simulink model "plant"  (R2026a)
settings: Solver=VariableStepAuto  StopTime=11
InitFcn:
  | run('plant_parameters.m');
values from neighbouring files (symbols this model uses):
  d = 0.1845    [plant_parameters.m]
  dd = d / sqrt(2)    [plant_parameters.m]
  Kd_J1 = 40    [plant_parameters.m]
  Kd_J2 = 30    [plant_parameters.m]
  Kd_J3 = 12    [plant_parameters.m]
  Ki_J1 = 800    [plant_parameters.m]
  Ki_J2 = 700    [plant_parameters.m]
  Ki_J3 = 300    [plant_parameters.m]
  Kp_J1 = 800    [plant_parameters.m]
  Kp_J2 = 600    [plant_parameters.m]
  Kp_J3 = 250    [plant_parameters.m]
  L1 = 0.074    [plant_parameters.m]
  L2 = 0.121    [plant_parameters.m]
  L3 = 0.230    (= 0.23)    [plant_parameters.m]
  N_J1 = 120    [plant_parameters.m]
  N_J2 = 120    [plant_parameters.m]
  N_J3 = 120    [plant_parameters.m]
  Sampling_Time = 0.005    [plant_parameters.m]
undefined symbols (not defined in the file or in its folder): X, Y, Z
libraries: sm_lib x121, nesl_utility x55, slpidlib x18
(part 1 of 8)
settings Model: Creator=bogon  LastModifiedBy=bogon

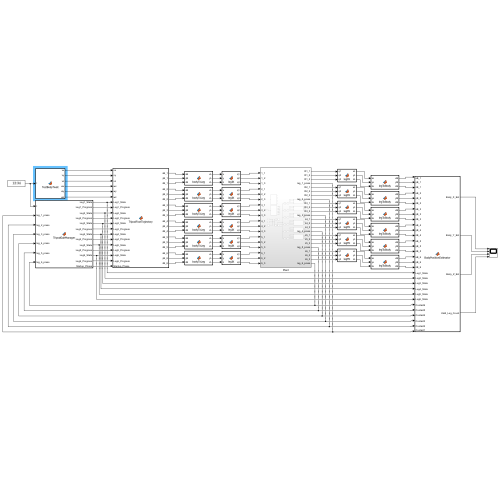
[thumbnail: Simulink's stored preview of the top-level diagram]
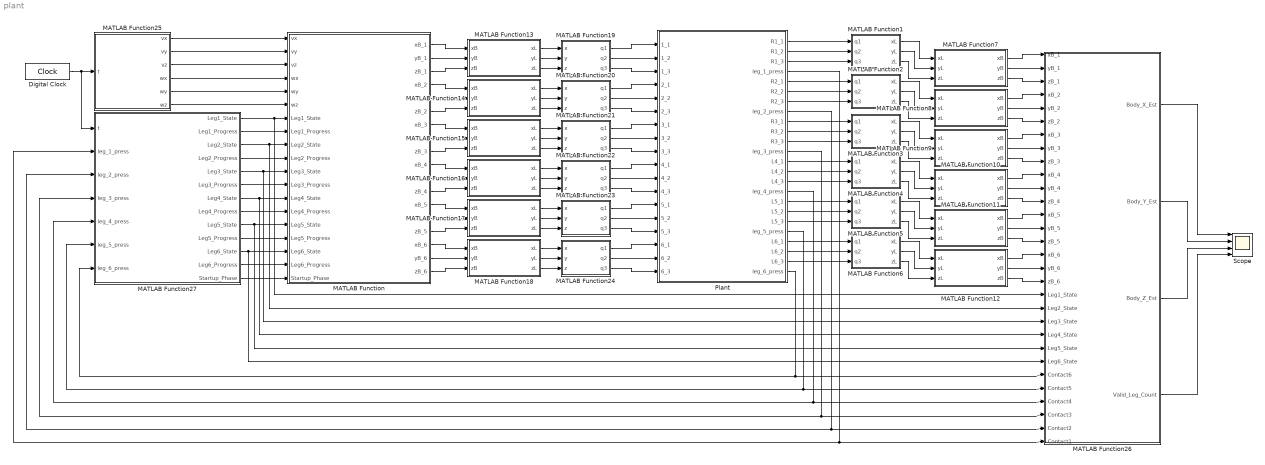
== system plant ==
  Digital Clock : DigitalClock  SampleTime=Sampling_Time
  MATLAB Function : MATLAB Function  TreatAsAtomicUnit=on
  MATLAB Function1 : MATLAB Function  TreatAsAtomicUnit=on
  MATLAB Function10 : MATLAB Function  TreatAsAtomicUnit=on
  MATLAB Function11 : MATLAB Function  TreatAsAtomicUnit=on
  MATLAB Function12 : MATLAB Function  TreatAsAtomicUnit=on
  MATLAB Function13 : MATLAB Function  TreatAsAtomicUnit=on
  MATLAB Function14 : MATLAB Function  TreatAsAtomicUnit=on
  MATLAB Function15 : MATLAB Function  TreatAsAtomicUnit=on
  MATLAB Function16 : MATLAB Function  TreatAsAtomicUnit=on
  MATLAB Function17 : MATLAB Function  TreatAsAtomicUnit=on
  MATLAB Function18 : MATLAB Function  TreatAsAtomicUnit=on
  MATLAB Function19 : MATLAB Function  TreatAsAtomicUnit=on
  MATLAB Function2 : MATLAB Function  TreatAsAtomicUnit=on
  MATLAB Function20 : MATLAB Function  TreatAsAtomicUnit=on
  MATLAB Function21 : MATLAB Function  TreatAsAtomicUnit=on
  MATLAB Function22 : MATLAB Function  TreatAsAtomicUnit=on
  MATLAB Function23 : MATLAB Function  TreatAsAtomicUnit=on
  MATLAB Function24 : MATLAB Function  TreatAsAtomicUnit=on
  MATLAB Function25 : MATLAB Function  TreatAsAtomicUnit=on
  MATLAB Function26 : MATLAB Function  TreatAsAtomicUnit=on  SystemSampleTime=Sampling_Time
  MATLAB Function27 : MATLAB Function  TreatAsAtomicUnit=on
  MATLAB Function3 : MATLAB Function  TreatAsAtomicUnit=on
  MATLAB Function4 : MATLAB Function  TreatAsAtomicUnit=on
  MATLAB Function5 : MATLAB Function  TreatAsAtomicUnit=on
  MATLAB Function6 : MATLAB Function  TreatAsAtomicUnit=on
  MATLAB Function7 : MATLAB Function  TreatAsAtomicUnit=on
  MATLAB Function8 : MATLAB Function  TreatAsAtomicUnit=on
  MATLAB Function9 : MATLAB Function  TreatAsAtomicUnit=on
  Plant : Subsystem
  Scope : Scope  NumInputPorts=4
      settings: ActiveDisplayYMinimum=-3.1042012313067247  ActiveDisplayYMaximum=1.7303656403267551
  wires:
  Plant/1(R1_1) -> MATLAB Function1/1(q1)
  Plant/2(R1_2) -> MATLAB Function1/2(q2)
  Plant/3(R1_3) -> MATLAB Function1/3(q3)
  Plant/9(R3_1) -> MATLAB Function3/1(q1)
  Plant/10(R3_2) -> MATLAB Function3/2(q2)
  Plant/11(R3_3) -> MATLAB Function3/3(q3)
  Plant/5(R2_1) -> MATLAB Function2/1(q1)
  Plant/6(R2_2) -> MATLAB Function2/2(q2)
  Plant/7(R2_3) -> MATLAB Function2/3(q3)
  Plant/13(L4_1) -> MATLAB Function4/1(q1)
  Plant/14(L4_2) -> MATLAB Function4/2(q2)
  Plant/15(L4_3) -> MATLAB Function4/3(q3)
  Plant/17(L5_1) -> MATLAB Function5/1(q1)
  Plant/18(L5_2) -> MATLAB Function5/2(q2)
  Plant/19(L5_3) -> MATLAB Function5/3(q3)
  Plant/21(L6_1) -> MATLAB Function6/1(q1)
  Plant/22(L6_2) -> MATLAB Function6/2(q2)
  Plant/23(L6_3) -> MATLAB Function6/3(q3)
  MATLAB Function16/1(xL) -> MATLAB Function22/1(x)
  MATLAB Function16/3(zL) -> MATLAB Function22/3(z)
  MATLAB Function16/2(yL) -> MATLAB Function22/2(y)
  MATLAB Function18/1(xL) -> MATLAB Function24/1(x)
  MATLAB Function17/3(zL) -> MATLAB Function23/3(z)
  MATLAB Function17/1(xL) -> MATLAB Function23/1(x)
  MATLAB Function18/2(yL) -> MATLAB Function24/2(y)
  MATLAB Function17/2(yL) -> MATLAB Function23/2(y)
  MATLAB Function14/3(zL) -> MATLAB Function20/3(z)
  MATLAB Function13/2(yL) -> MATLAB Function19/2(y)
  MATLAB Function15/3(zL) -> MATLAB Function21/3(z)
  MATLAB Function18/3(zL) -> MATLAB Function24/3(z)
  MATLAB Function/14(yB_5) -> MATLAB Function17/2(yB)
  MATLAB Function15/2(yL) -> MATLAB Function21/2(y)
  MATLAB Function/18(zB_6) -> MATLAB Function18/3(zB)
  MATLAB Function/5(yB_2) -> MATLAB Function14/2(yB)
  MATLAB Function/16(xB_6) -> MATLAB Function18/1(xB)
  MATLAB Function/17(yB_6) -> MATLAB Function18/2(yB)
  MATLAB Function/6(zB_2) -> MATLAB Function14/3(zB)
  MATLAB Function/11(yB_4) -> MATLAB Function16/2(yB)
  MATLAB Function/13(xB_5) -> MATLAB Function17/1(xB)
  MATLAB Function/8(yB_3) -> MATLAB Function15/2(yB)
  MATLAB Function/15(zB_5) -> MATLAB Function17/3(zB)
  MATLAB Function14/1(xL) -> MATLAB Function20/1(x)
  MATLAB Function/10(xB_4) -> MATLAB Function16/1(xB)
  MATLAB Function/4(xB_2) -> MATLAB Function14/1(xB)
  MATLAB Function/9(zB_3) -> MATLAB Function15/3(zB)
  MATLAB Function14/2(yL) -> MATLAB Function20/2(y)
  MATLAB Function/12(zB_4) -> MATLAB Function16/3(zB)
  MATLAB Function/7(xB_3) -> MATLAB Function15/1(xB)
  MATLAB Function13/3(zL) -> MATLAB Function19/3(z)
  MATLAB Function15/1(xL) -> MATLAB Function21/1(x)
  MATLAB Function13/1(xL) -> MATLAB Function19/1(x)
  MATLAB Function19/1(q1) -> Plant/1(1_1)
  MATLAB Function19/2(q2) -> Plant/2(1_2)
  MATLAB Function19/3(q3) -> Plant/3(1_3)
  MATLAB Function20/2(q2) -> Plant/5(2_2)
  MATLAB Function20/1(q1) -> Plant/4(2_1)
  MATLAB Function20/3(q3) -> Plant/6(2_3)
  MATLAB Function21/1(q1) -> Plant/7(3_1)
  MATLAB Function21/2(q2) -> Plant/8(3_2)
  MATLAB Function21/3(q3) -> Plant/9(3_3)
  MATLAB Function22/1(q1) -> Plant/10(4_1)
  MATLAB Function22/2(q2) -> Plant/11(4_2)
  MATLAB Function22/3(q3) -> Plant/12(4_3)
  MATLAB Function23/1(q1) -> Plant/13(5_1)
  MATLAB Function23/2(q2) -> Plant/14(5_2)
  MATLAB Function23/3(q3) -> Plant/15(5_3)
  MATLAB Function24/2(q2) -> Plant/17(6_2)
  MATLAB Function24/1(q1) -> Plant/16(6_1)
  MATLAB Function24/3(q3) -> Plant/18(6_3)
  MATLAB Function1/1(xL) -> MATLAB Function7/1(xL)
  MATLAB Function1/2(yL) -> MATLAB Function7/2(yL)
  MATLAB Function1/3(zL) -> MATLAB Function7/3(zL)
  MATLAB Function2/1(xL) -> MATLAB Function8/1(xL)
  MATLAB Function2/2(yL) -> MATLAB Function8/2(yL)
  MATLAB Function2/3(zL) -> MATLAB Function8/3(zL)
  MATLAB Function3/1(xL) -> MATLAB Function9/1(xL)
  MATLAB Function3/2(yL) -> MATLAB Function9/2(yL)
  MATLAB Function3/3(zL) -> MATLAB Function9/3(zL)
  MATLAB Function4/1(xL) -> MATLAB Function10/1(xL)
  MATLAB Function4/2(yL) -> MATLAB Function10/2(yL)
  MATLAB Function4/3(zL) -> MATLAB Function10/3(zL)
  MATLAB Function5/1(xL) -> MATLAB Function11/1(xL)
  MATLAB Function5/2(yL) -> MATLAB Function11/2(yL)
  MATLAB Function5/3(zL) -> MATLAB Function11/3(zL)
  MATLAB Function6/1(xL) -> MATLAB Function12/1(xL)
  MATLAB Function6/2(yL) -> MATLAB Function12/2(yL)
  MATLAB Function6/3(zL) -> MATLAB Function12/3(zL)
  Digital Clock/1 -> MATLAB Function27/1(t), MATLAB Function25/1(t)
  MATLAB Function/1(xB_1) -> MATLAB Function13/1(xB)
  MATLAB Function/2(yB_1) -> MATLAB Function13/2(yB)
  MATLAB Function/3(zB_1) -> MATLAB Function13/3(zB)
  MATLAB Function25/1(vx) -> MATLAB Function/1(vx)
  MATLAB Function25/2(vy) -> MATLAB Function/2(vy)
  MATLAB Function25/3(vz) -> MATLAB Function/3(vz)
  MATLAB Function25/4(wx) -> MATLAB Function/4(wx)
  MATLAB Function25/5(wy) -> MATLAB Function/5(wy)
  MATLAB Function25/6(wz) -> MATLAB Function/6(wz)
  MATLAB Function27/1(Leg1_State) -> MATLAB Function26/19(Leg1_State), MATLAB Function/7(Leg1_State)
  MATLAB Function27/2(Leg1_Progress) -> MATLAB Function/8(Leg1_Progress)
  MATLAB Function27/3(Leg2_State) -> MATLAB Function26/20(Leg2_State), MATLAB Function/9(Leg2_State)
  MATLAB Function27/4(Leg2_Progress) -> MATLAB Function/10(Leg2_Progress)
  MATLAB Function27/5(Leg3_State) -> MATLAB Function26/21(Leg3_State), MATLAB Function/11(Leg3_State)
  MATLAB Function27/6(Leg3_Progress) -> MATLAB Function/12(Leg3_Progress)
  MATLAB Function27/7(Leg4_State) -> MATLAB Function26/22(Leg4_State), MATLAB Function/13(Leg4_State)
  MATLAB Function27/8(Leg4_Progress) -> MATLAB Function/14(Leg4_Progress)
  MATLAB Function27/9(Leg5_State) -> MATLAB Function26/23(Leg5_State), MATLAB Function/15(Leg5_State)
  MATLAB Function27/10(Leg5_Progress) -> MATLAB Function/16(Leg5_Progress)
  MATLAB Function27/11(Leg6_State) -> MATLAB Function26/24(Leg6_State), MATLAB Function/17(Leg6_State)
  MATLAB Function27/12(Leg6_Progress) -> MATLAB Function/18(Leg6_Progress)
  MATLAB Function27/13(Startup_Phase) -> MATLAB Function/19(Startup_Phase)
  Plant/4(leg_1_press) -> MATLAB Function26/30(Contact1), MATLAB Function27/2(leg_1_press)
  Plant/8(leg_2_press) -> MATLAB Function26/29(Contact2), MATLAB Function27/3(leg_2_press)
  Plant/12(leg_3_press) -> MATLAB Function27/4(leg_3_press), MATLAB Function26/28(Contact3)
  Plant/16(leg_4_press) -> MATLAB Function26/27(Contact4), MATLAB Function27/5(leg_4_press)
  Plant/20(leg_5_press) -> MATLAB Function27/6(leg_5_press), MATLAB Function26/26(Contact5)
  Plant/24(leg_6_press) -> MATLAB Function27/7(leg_6_press), MATLAB Function26/25(Contact6)
  MATLAB Function7/1(xB) -> MATLAB Function26/1(xB_1)
  MATLAB Function7/2(yB) -> MATLAB Function26/2(yB_1)
  MATLAB Function7/3(zB) -> MATLAB Function26/3(zB_1)
  MATLAB Function12/3(zB) -> MATLAB Function26/18(zB_6)
  MATLAB Function12/2(yB) -> MATLAB Function26/17(yB_6)
  MATLAB Function12/1(xB) -> MATLAB Function26/16(xB_6)
  MATLAB Function8/2(yB) -> MATLAB Function26/5(yB_2)
  MATLAB Function9/2(yB) -> MATLAB Function26/8(yB_3)
  MATLAB Function10/2(yB) -> MATLAB Function26/11(yB_4)
  MATLAB Function11/2(yB) -> MATLAB Function26/14(yB_5)
  MATLAB Function11/3(zB) -> MATLAB Function26/15(zB_5)
  MATLAB Function11/1(xB) -> MATLAB Function26/13(xB_5)
  MATLAB Function10/3(zB) -> MATLAB Function26/12(zB_4)
  MATLAB Function10/1(xB) -> MATLAB Function26/10(xB_4)
  MATLAB Function9/3(zB) -> MATLAB Function26/9(zB_3)
  MATLAB Function9/1(xB) -> MATLAB Function26/7(xB_3)
  MATLAB Function8/3(zB) -> MATLAB Function26/6(zB_2)
  MATLAB Function8/1(xB) -> MATLAB Function26/4(xB_2)
  MATLAB Function26/1(Body_X_Est) -> Scope/1
  MATLAB Function26/2(Body_Y_Est) -> Scope/2
  MATLAB Function26/3(Body_Z_Est) -> Scope/3
  MATLAB Function26/4(Valid_Leg_Count) -> Scope/4

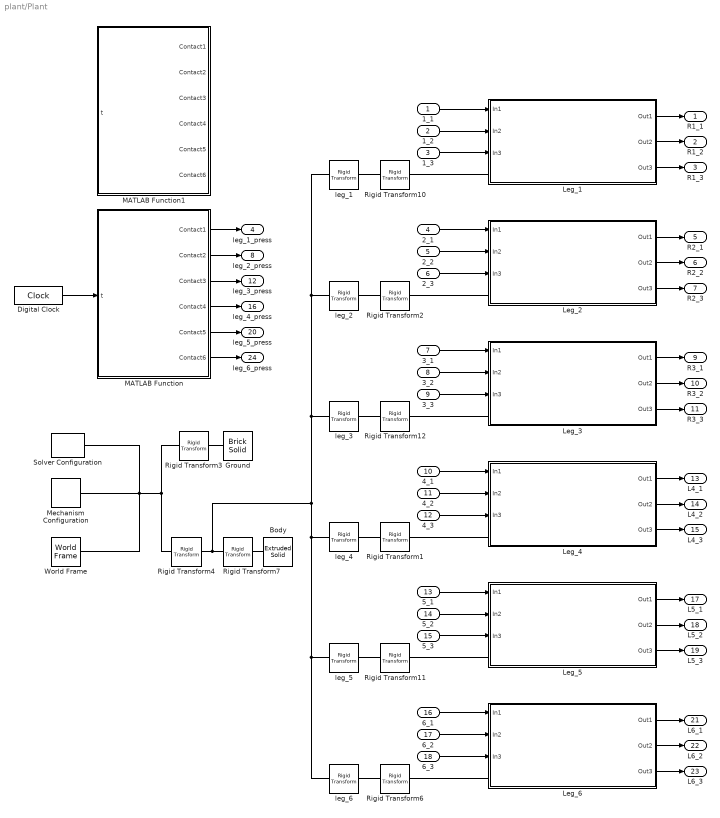
== system plant/Plant ==
  1_1 : Inport
  1_2 : Inport  Port=2
  1_3 : Inport  Port=3
  2_1 : Inport  Port=4
  2_2 : Inport  Port=5
  2_3 : Inport  Port=6
  3_1 : Inport  Port=7
  3_2 : Inport  Port=8
  3_3 : Inport  Port=9
  4_1 : Inport  Port=10
  4_2 : Inport  Port=11
  4_3 : Inport  Port=12
  5_1 : Inport  Port=13
  5_2 : Inport  Port=14
  5_3 : Inport  Port=15
  6_1 : Inport  Port=16
  6_2 : Inport  Port=17
  6_3 : Inport  Port=18
  Body : sm_lib/Body Elements/Extruded Solid  ExtrusionType=Regular  PolygonNumSides=8  PolygonOuterRadius=Body_r  PolygonOuterRadiusUnits=m  ExportEntireGeometry=off  ExtrusionCrossSection=[1 1; -1 1; -1 -1; 1 -1]  ExtrusionCrossSectionUnits=m  ExportConvexHullGeometry=off  ExtrusionLength=Body_t  ExtrusionLengthUnits=m  InertiaType=CalculateFromGeometry  BasedOnType=Density  Density=1000  DensityUnits=kg/m^3  Mass=1  MassUnits=kg  CenterOfMass=[0 0 0]  CenterOfMassUnits=m  MomentsOfInertia=[1 1 1]  MomentsOfInertiaUnits=kg*m^2  ProductsOfInertia=[0 0 0]  ProductsOfInertiaUnits=kg*m^2  GraphicType=FromGeometry  MarkerShape=Sphere  MarkerSize=10  GraphicVisPropType=SimpleVisualProperties  GraphicDiffuseColor=[0 0 0]  GraphicOpacity=1  GraphicSpecularColor=[0.5 0.5 0.5 1.0]  GraphicAmbientColor=[0.15 0.15 0.15 1.0]  GraphicEmissiveColor=[0.0 0.0 0.0 1.0]  GraphicShininess=75  DoExposeReferenceFrame=on  SerializedFrames=<Frames/>
  Digital Clock : DigitalClock  SampleTime=Sampling_Time
  Ground : sm_lib/Body Elements/Brick Solid  BrickDimensions=[2 2 0.05]  BrickDimensionsUnits=m  ExportEntireGeometry=off  InertiaType=CalculateFromGeometry  BasedOnType=Density  Density=1000  DensityUnits=kg/m^3  Mass=1  MassUnits=kg  CenterOfMass=[0 0 0]  CenterOfMassUnits=m  MomentsOfInertia=[1 1 1]  MomentsOfInertiaUnits=kg*m^2  ProductsOfInertia=[0 0 0]  ProductsOfInertiaUnits=kg*m^2  GraphicType=FromGeometry  MarkerShape=Sphere  MarkerSize=10  GraphicVisPropType=SimpleVisualProperties  GraphicDiffuseColor=[0 1 0.498]  GraphicOpacity=1  GraphicSpecularColor=[0.5 0.5 0.5 1.0]  GraphicAmbientColor=[0.15 0.15 0.15 1.0]  GraphicEmissiveColor=[0.0 0.0 0.0 1.0]  GraphicShininess=75  DoExposeReferenceFrame=on  SerializedFrames=<Frames/>
  Leg_1 : Subsystem
  Leg_2 : Subsystem
  Leg_3 : Subsystem
  Leg_4 : Subsystem
  Leg_5 : Subsystem
  Leg_6 : Subsystem
  MATLAB Function : MATLAB Function  TreatAsAtomicUnit=on
  MATLAB Function1 : MATLAB Function  TreatAsAtomicUnit=on
  Mechanism Configuration : sm_lib/Utilities/Mechanism Configuration  UniformGravity=Constant  GravityVector=[0 0 -9.80665]  GravityVectorUnits=m/s^2  LinearizationDelta=0.001  JointModeTransitionNonlinearIterations=2
  Rigid Transform1 : sm_lib/Frames and Transforms/Rigid Transform  RotationMethod=StandardAxis  FollAlignAxisA=+X  BaseAlignAxisA=+Y  FollAlignAxisB=+Y  BaseAlignAxisB=+Z  RotationStandardAxis=+Z  RotationAngle=45  RotationAngleUnits=deg  RotationArbitraryAxis=[0 0 1]  RotationSequenceAxes=FollowerAxes  RotationSequence=XYX  RotationSequenceAngles=[0 0 0]  RotationSequenceAnglesUnits=deg  RotationMatrix=[1 0 0;0 1 0;0 0 1]  Quaternion=[1 0 0 0]  TranslationMethod=None  TranslationCartesianOffset=[0 0 -0.025]  TranslationCartesianOffsetUnits=m  TranslationStandardAxis=-Z  TranslationStandardOffset=0.025  TranslationStandardOffsetUnits=m  TranslationROffset=0  TranslationROffsetUnits=m  TranslationThetaOffset=0  TranslationThetaOffsetUnits=deg  TranslationZOffset=0  TranslationZOffsetUnits=m
  Rigid Transform10 : sm_lib/Frames and Transforms/Rigid Transform  RotationMethod=StandardAxis  FollAlignAxisA=+X  BaseAlignAxisA=+Y  FollAlignAxisB=+Y  BaseAlignAxisB=+Z  RotationStandardAxis=-Z  RotationAngle=45  RotationAngleUnits=deg  RotationArbitraryAxis=[0 0 1]  RotationSequenceAxes=FollowerAxes  RotationSequence=XYX  RotationSequenceAngles=[0 0 0]  RotationSequenceAnglesUnits=deg  RotationMatrix=[1 0 0;0 1 0;0 0 1]  Quaternion=[1 0 0 0]  TranslationMethod=None  TranslationCartesianOffset=[0 0 -0.025]  TranslationCartesianOffsetUnits=m  TranslationStandardAxis=-Z  TranslationStandardOffset=0.025  TranslationStandardOffsetUnits=m  TranslationROffset=0  TranslationROffsetUnits=m  TranslationThetaOffset=0  TranslationThetaOffsetUnits=deg  TranslationZOffset=0  TranslationZOffsetUnits=m
  Rigid Transform11 : sm_lib/Frames and Transforms/Rigid Transform  RotationMethod=StandardAxis  FollAlignAxisA=+X  BaseAlignAxisA=+Y  FollAlignAxisB=+Y  BaseAlignAxisB=+Z  RotationStandardAxis=+Z  RotationAngle=90  RotationAngleUnits=deg  RotationArbitraryAxis=[0 0 1]  RotationSequenceAxes=FollowerAxes  RotationSequence=XYX  RotationSequenceAngles=[0 0 0]  RotationSequenceAnglesUnits=deg  RotationMatrix=[1 0 0;0 1 0;0 0 1]  Quaternion=[1 0 0 0]  TranslationMethod=None  TranslationCartesianOffset=[0 0 -0.025]  TranslationCartesianOffsetUnits=m  TranslationStandardAxis=-Z  TranslationStandardOffset=0.025  TranslationStandardOffsetUnits=m  TranslationROffset=0  TranslationROffsetUnits=m  TranslationThetaOffset=0  TranslationThetaOffsetUnits=deg  TranslationZOffset=0  TranslationZOffsetUnits=m
  Rigid Transform12 : sm_lib/Frames and Transforms/Rigid Transform  RotationMethod=StandardAxis  FollAlignAxisA=+X  BaseAlignAxisA=+Y  FollAlignAxisB=+Y  BaseAlignAxisB=+Z  RotationStandardAxis=-Z  RotationAngle=135  RotationAngleUnits=deg  RotationArbitraryAxis=[0 0 1]  RotationSequenceAxes=BaseAxes  RotationSequence=XYX  RotationSequenceAngles=[0 0 0]  RotationSequenceAnglesUnits=deg  RotationMatrix=[1 0 0;0 1 0;0 0 1]  Quaternion=[1 0 0 0]  TranslationMethod=None  TranslationCartesianOffset=[0 0 -0.025]  TranslationCartesianOffsetUnits=m  TranslationStandardAxis=-Z  TranslationStandardOffset=0.025  TranslationStandardOffsetUnits=m  TranslationROffset=0  TranslationROffsetUnits=m  TranslationThetaOffset=0  TranslationThetaOffsetUnits=deg  TranslationZOffset=0  TranslationZOffsetUnits=m
  Rigid Transform2 : sm_lib/Frames and Transforms/Rigid Transform  RotationMethod=StandardAxis  FollAlignAxisA=+X  BaseAlignAxisA=+Y  FollAlignAxisB=+Y  BaseAlignAxisB=+Z  RotationStandardAxis=-Z  RotationAngle=90  RotationAngleUnits=deg  RotationArbitraryAxis=[0 0 1]  RotationSequenceAxes=FollowerAxes  RotationSequence=XYX  RotationSequenceAngles=[0 0 0]  RotationSequenceAnglesUnits=deg  RotationMatrix=[1 0 0;0 1 0;0 0 1]  Quaternion=[1 0 0 0]  TranslationMethod=None  TranslationCartesianOffset=[0 0 -0.025]  TranslationCartesianOffsetUnits=m  TranslationStandardAxis=-Z  TranslationStandardOffset=0.025  TranslationStandardOffsetUnits=m  TranslationROffset=0  TranslationROffsetUnits=m  TranslationThetaOffset=0  TranslationThetaOffsetUnits=deg  TranslationZOffset=0  TranslationZOffsetUnits=m
  Rigid Transform3 : sm_lib/Frames and Transforms/Rigid Transform  RotationMethod=None  FollAlignAxisA=+X  BaseAlignAxisA=+Y  FollAlignAxisB=+Y  BaseAlignAxisB=+Z  RotationStandardAxis=+Z  RotationAngle=0  RotationAngleUnits=deg  RotationArbitraryAxis=[0 0 1]  RotationSequenceAxes=FollowerAxes  RotationSequence=XYX  RotationSequenceAngles=[0 0 0]  RotationSequenceAnglesUnits=deg  RotationMatrix=[1 0 0;0 1 0;0 0 1]  Quaternion=[1 0 0 0]  TranslationMethod=Cartesian  TranslationCartesianOffset=[0 0 -0.025]  TranslationCartesianOffsetUnits=m  TranslationStandardAxis=-Z  TranslationStandardOffset=0.025  TranslationStandardOffsetUnits=m  TranslationROffset=0  TranslationROffsetUnits=m  TranslationThetaOffset=0  TranslationThetaOffsetUnits=deg  TranslationZOffset=0  TranslationZOffsetUnits=m
  Rigid Transform4 : sm_lib/Frames and Transforms/Rigid Transform  RotationMethod=None  FollAlignAxisA=+X  BaseAlignAxisA=+Y  FollAlignAxisB=+Y  BaseAlignAxisB=+Z  RotationStandardAxis=+Z  RotationAngle=90  RotationAngleUnits=deg  RotationArbitraryAxis=[0 0 1]  RotationSequenceAxes=FollowerAxes  RotationSequence=XYX  RotationSequenceAngles=[0 0 0]  RotationSequenceAnglesUnits=deg  RotationMatrix=[1 0 0;0 1 0;0 0 1]  Quaternion=[1 0 0 0]  TranslationMethod=StandardAxis  TranslationCartesianOffset=[0 0 0]  TranslationCartesianOffsetUnits=m  TranslationStandardAxis=+Z  TranslationStandardOffset=Reference_point  TranslationStandardOffsetUnits=m  TranslationROffset=0  TranslationROffsetUnits=m  TranslationThetaOffset=0  TranslationThetaOffsetUnits=deg  TranslationZOffset=0  TranslationZOffsetUnits=m
  Rigid Transform6 : sm_lib/Frames and Transforms/Rigid Transform  RotationMethod=StandardAxis  FollAlignAxisA=+X  BaseAlignAxisA=+Y  FollAlignAxisB=+Y  BaseAlignAxisB=+Z  RotationStandardAxis=+Z  RotationAngle=135  RotationAngleUnits=deg  RotationArbitraryAxis=[0 0 1]  RotationSequenceAxes=FollowerAxes  RotationSequence=XYX  RotationSequenceAngles=[0 0 0]  RotationSequenceAnglesUnits=deg  RotationMatrix=[1 0 0;0 1 0;0 0 1]  Quaternion=[1 0 0 0]  TranslationMethod=None  TranslationCartesianOffset=[0 0 -0.025]  TranslationCartesianOffsetUnits=m  TranslationStandardAxis=-Z  TranslationStandardOffset=0.025  TranslationStandardOffsetUnits=m  TranslationROffset=0  TranslationROffsetUnits=m  TranslationThetaOffset=0  TranslationThetaOffsetUnits=deg  TranslationZOffset=0  TranslationZOffsetUnits=m
  Rigid Transform7 : sm_lib/Frames and Transforms/Rigid Transform  RotationMethod=StandardAxis  FollAlignAxisA=+X  BaseAlignAxisA=+Y  FollAlignAxisB=+Y  BaseAlignAxisB=+Z  RotationStandardAxis=-Z  RotationAngle=22.5  RotationAngleUnits=deg  RotationArbitraryAxis=[0 0 1]  RotationSequenceAxes=FollowerAxes  RotationSequence=XYX  RotationSequenceAngles=[0 0 0]  RotationSequenceAnglesUnits=deg  RotationMatrix=[1 0 0;0 1 0;0 0 1]  Quaternion=[1 0 0 0]  TranslationMethod=None  TranslationCartesianOffset=[0 0 -0.025]  TranslationCartesianOffsetUnits=m  TranslationStandardAxis=+Y  TranslationStandardOffset=0.025  TranslationStandardOffsetUnits=m  TranslationROffset=0  TranslationROffsetUnits=m  TranslationThetaOffset=0  TranslationThetaOffsetUnits=deg  TranslationZOffset=0  TranslationZOffsetUnits=m
  Solver Configuration : nesl_utility/Solver Configuration  PhysicalDomain=network_engine_domain  SubClassName=solver  LeftPortType=input  RightPortType=generic  Tones=[]  Harmonics=[]  SimulateNoise=off  Profile=off  UseLocalSampling=off  EnableSwitchedLinearOptims=on  FrequencyDomain=off  UseCCode=off  RelTol=0.001  AbsTol=0.001  MinStep=1e-09  ToWorkspace=off  RevertToSquareIcSolve=off  NumHomotopyIterations=100  PhasorMode=off  PhasorModeNumHarmonics=1  ConsistencySolver=NEWTON_XTOL_AFTER_FTOL  CanonicalOrdering=CANONICAL  OptimizeIntermediates=OPTIMIZED  IndexReductionMethod=DerivativeReplacement  DoDC=off  ResidualTolerance=1e-09  ConsistencyTolSource=GLOBAL  ConsistencyAbsTol=0.001  ConsistencyRelTol=0.001  ConsistencyTolFactor=0.001  UseLocalSolver=off  LocalSolverChoice=NE_BACKWARD_EULER_ADVANCER  ResolveIndetEquations=on  FunctionEvalNumThread=1  LocalSolverSampleTime=0.001  DoFixedCost=off  MaxNonlinIter=3  MaxModeIter=2  ComputeImpulses=off  ImpulseIterations=2  LinearAlgebra=auto  LinearAlgebraNumThread=0  EquationFormulation=NE_TIME_EF  DelaysMemoryBudget=1024  AutomaticFiltering=on  FilteringTimeConstant=0.001  PartitionStorageMethod=AS_NEEDED  PartitionMemoryBudget=1024  PartitionMethod=ROBUST  MultibodyUseLocalSolver=off  MultibodyLocalSolverChoice=ODE1  MultibodyLocalSolverSampleTime=0.001
  World Frame : sm_lib/Frames and Transforms/World Frame
  leg_1 : sm_lib/Frames and Transforms/Rigid Transform  RotationMethod=None  FollAlignAxisA=+X  BaseAlignAxisA=+Y  FollAlignAxisB=+Y  BaseAlignAxisB=+Z  RotationStandardAxis=+Z  RotationAngle=0  RotationAngleUnits=deg  RotationArbitraryAxis=[0 0 1]  RotationSequenceAxes=FollowerAxes  RotationSequence=XYX  RotationSequenceAngles=[0 0 0]  RotationSequenceAnglesUnits=deg  RotationMatrix=[1 0 0;0 1 0;0 0 1]  Quaternion=[1 0 0 0]  TranslationMethod=Cartesian  TranslationCartesianOffset=[dd -dd 0]  TranslationCartesianOffsetUnits=m  TranslationStandardAxis=-Z  TranslationStandardOffset=0.025  TranslationStandardOffsetUnits=m  TranslationROffset=0  TranslationROffsetUnits=m  TranslationThetaOffset=0  TranslationThetaOffsetUnits=deg  TranslationZOffset=0  TranslationZOffsetUnits=m
  leg_2 : sm_lib/Frames and Transforms/Rigid Transform  RotationMethod=None  FollAlignAxisA=+X  BaseAlignAxisA=+Y  FollAlignAxisB=+Y  BaseAlignAxisB=+Z  RotationStandardAxis=+Z  RotationAngle=0  RotationAngleUnits=deg  RotationArbitraryAxis=[0 0 1]  RotationSequenceAxes=FollowerAxes  RotationSequence=XYX  RotationSequenceAngles=[0 0 0]  RotationSequenceAnglesUnits=deg  RotationMatrix=[1 0 0;0 1 0;0 0 1]  Quaternion=[1 0 0 0]  TranslationMethod=Cartesian  TranslationCartesianOffset=[0 -d 0]  TranslationCartesianOffsetUnits=m  TranslationStandardAxis=-Z  TranslationStandardOffset=0.025  TranslationStandardOffsetUnits=m  TranslationROffset=0  TranslationROffsetUnits=m  TranslationThetaOffset=0  TranslationThetaOffsetUnits=deg  TranslationZOffset=0  TranslationZOffsetUnits=m
  leg_3 : sm_lib/Frames and Transforms/Rigid Transform  RotationMethod=None  FollAlignAxisA=+X  BaseAlignAxisA=+Y  FollAlignAxisB=+Y  BaseAlignAxisB=+Z  RotationStandardAxis=+Z  RotationAngle=0  RotationAngleUnits=deg  RotationArbitraryAxis=[0 0 1]  RotationSequenceAxes=FollowerAxes  RotationSequence=XYX  RotationSequenceAngles=[0 0 0]  RotationSequenceAnglesUnits=deg  RotationMatrix=[1 0 0;0 1 0;0 0 1]  Quaternion=[1 0 0 0]  TranslationMethod=Cartesian  TranslationCartesianOffset=[-dd -dd 0]  TranslationCartesianOffsetUnits=m  TranslationStandardAxis=-Z  TranslationStandardOffset=0.025  TranslationStandardOffsetUnits=m  TranslationROffset=0  TranslationROffsetUnits=m  TranslationThetaOffset=0  TranslationThetaOffsetUnits=deg  TranslationZOffset=0  TranslationZOffsetUnits=m
  leg_4 : sm_lib/Frames and Transforms/Rigid Transform  RotationMethod=None  FollAlignAxisA=+X  BaseAlignAxisA=+Y  FollAlignAxisB=+Y  BaseAlignAxisB=+Z  RotationStandardAxis=+Z  RotationAngle=0  RotationAngleUnits=deg  RotationArbitraryAxis=[0 0 1]  RotationSequenceAxes=FollowerAxes  RotationSequence=XYX  RotationSequenceAngles=[0 0 0]  RotationSequenceAnglesUnits=deg  RotationMatrix=[1 0 0;0 1 0;0 0 1]  Quaternion=[1 0 0 0]  TranslationMethod=Cartesian  TranslationCartesianOffset=[dd dd 0]  TranslationCartesianOffsetUnits=m  TranslationStandardAxis=-Z  TranslationStandardOffset=0.025  TranslationStandardOffsetUnits=m  TranslationROffset=0  TranslationROffsetUnits=m  TranslationThetaOffset=0  TranslationThetaOffsetUnits=deg  TranslationZOffset=0  TranslationZOffsetUnits=m
  leg_5 : sm_lib/Frames and Transforms/Rigid Transform  RotationMethod=None  FollAlignAxisA=+X  BaseAlignAxisA=+Y  FollAlignAxisB=+Y  BaseAlignAxisB=+Z  RotationStandardAxis=+Z  RotationAngle=0  RotationAngleUnits=deg  RotationArbitraryAxis=[0 0 1]  RotationSequenceAxes=FollowerAxes  RotationSequence=XYX  RotationSequenceAngles=[0 0 0]  RotationSequenceAnglesUnits=deg  RotationMatrix=[1 0 0;0 1 0;0 0 1]  Quaternion=[1 0 0 0]  TranslationMethod=Cartesian  TranslationCartesianOffset=[0 d 0]  TranslationCartesianOffsetUnits=m  TranslationStandardAxis=-Z  TranslationStandardOffset=0.025  TranslationStandardOffsetUnits=m  TranslationROffset=0  TranslationROffsetUnits=m  TranslationThetaOffset=0  TranslationThetaOffsetUnits=deg  TranslationZOffset=0  TranslationZOffsetUnits=m
  leg_6 : sm_lib/Frames and Transforms/Rigid Transform  RotationMethod=None  FollAlignAxisA=+X  BaseAlignAxisA=+Y  FollAlignAxisB=+Y  BaseAlignAxisB=+Z  RotationStandardAxis=+Z  RotationAngle=0  RotationAngleUnits=deg  RotationArbitraryAxis=[0 0 1]  RotationSequenceAxes=FollowerAxes  RotationSequence=XYX  RotationSequenceAngles=[0 0 0]  RotationSequenceAnglesUnits=deg  RotationMatrix=[1 0 0;0 1 0;0 0 1]  Quaternion=[1 0 0 0]  TranslationMethod=Cartesian  TranslationCartesianOffset=[-dd dd 0]  TranslationCartesianOffsetUnits=m  TranslationStandardAxis=-Z  TranslationStandardOffset=0.025  TranslationStandardOffsetUnits=m  TranslationROffset=0  TranslationROffsetUnits=m  TranslationThetaOffset=0  TranslationThetaOffsetUnits=deg  TranslationZOffset=0  TranslationZOffsetUnits=m
  R1_1 : Outport
  R1_2 : Outport  Port=2
  R1_3 : Outport  Port=3
  leg_1_press : Outport  Port=4
  R2_1 : Outport  Port=5
  R2_2 : Outport  Port=6
  R2_3 : Outport  Port=7
  leg_2_press : Outport  Port=8
  R3_1 : Outport  Port=9
  R3_2 : Outport  Port=10
  R3_3 : Outport  Port=11
  leg_3_press : Outport  Port=12
  L4_1 : Outport  Port=13
  L4_2 : Outport  Port=14
  L4_3 : Outport  Port=15
  leg_4_press : Outport  Port=16
  L5_1 : Outport  Port=17
  L5_2 : Outport  Port=18
  L5_3 : Outport  Port=19
  leg_5_press : Outport  Port=20
  L6_1 : Outport  Port=21
  L6_2 : Outport  Port=22
  L6_3 : Outport  Port=23
  leg_6_press : Outport  Port=24
  wires:
  1_3/1 -> Leg_1/3(In3)
  4_1/1 -> Leg_4/1(In1)
  4_2/1 -> Leg_4/2(In2)
  6_3/1 -> Leg_6/3(In3)
  3_2/1 -> Leg_3/2(In2)
  6_1/1 -> Leg_6/1(In1)
  3_3/1 -> Leg_3/3(In3)
  1_2/1 -> Leg_1/2(In2)
  3_1/1 -> Leg_3/1(In1)
  4_3/1 -> Leg_4/3(In3)
  1_1/1 -> Leg_1/1(In1)
  6_2/1 -> Leg_6/2(In2)
  2_3/1 -> Leg_2/3(In3)
  2_1/1 -> Leg_2/1(In1)
  2_2/1 -> Leg_2/2(In2)
  5_3/1 -> Leg_5/3(In3)
  5_2/1 -> Leg_5/2(In2)
  5_1/1 -> Leg_5/1(In1)
  Leg_1/1(Out1) -> R1_1/1
  Leg_1/2(Out2) -> R1_2/1
  Leg_1/3(Out3) -> R1_3/1
  Leg_2/3(Out3) -> R2_3/1
  Leg_2/2(Out2) -> R2_2/1
  Leg_2/1(Out1) -> R2_1/1
  Leg_3/3(Out3) -> R3_3/1
  Leg_3/2(Out2) -> R3_2/1
  Leg_3/1(Out1) -> R3_1/1
  Leg_4/3(Out3) -> L4_3/1
  Leg_4/2(Out2) -> L4_2/1
  Leg_4/1(Out1) -> L4_1/1
  Leg_5/3(Out3) -> L5_3/1
  Leg_5/2(Out2) -> L5_2/1
  Leg_5/1(Out1) -> L5_1/1
  Leg_6/3(Out3) -> L6_3/1
  Leg_6/2(Out2) -> L6_2/1
  Leg_6/1(Out1) -> L6_1/1
  Digital Clock/1 -> MATLAB Function/1(t)
  MATLAB Function/2(Contact2) -> leg_2_press/1
  MATLAB Function/1(Contact1) -> leg_1_press/1
  MATLAB Function/3(Contact3) -> leg_3_press/1
  MATLAB Function/4(Contact4) -> leg_4_press/1
  MATLAB Function/5(Contact5) -> leg_5_press/1
  MATLAB Function/6(Contact6) -> leg_6_press/1
  connections:
  leg_4/RConn1 -- Rigid Transform1/LConn1
  Rigid Transform11/LConn1 -- leg_5/RConn1
  Rigid Transform4/LConn1 -- Rigid Transform3/LConn1 -- World Frame/RConn1 -- Mechanism Configuration/RConn1 -- Solver Configuration/RConn1
  Rigid Transform2/LConn1 -- leg_2/RConn1
  leg_6/RConn1 -- Rigid Transform6/LConn1
  Ground/RConn1 -- Rigid Transform3/RConn1
  leg_1/LConn1 -- leg_2/LConn1 -- leg_3/LConn1 -- Rigid Transform7/LConn1 -- Rigid Transform4/RConn1 -- leg_5/LConn1 -- leg_6/LConn1 -- leg_4/LConn1
  Leg_6/LConn1 -- Rigid Transform6/RConn1
  leg_3/RConn1 -- Rigid Transform12/LConn1
  Leg_4/LConn1 -- Rigid Transform1/RConn1
  Leg_3/LConn1 -- Rigid Transform12/RConn1
  leg_1/RConn1 -- Rigid Transform10/LConn1
  Rigid Transform10/RConn1 -- Leg_1/LConn1
  Leg_5/LConn1 -- Rigid Transform11/RConn1
  Leg_2/LConn1 -- Rigid Transform2/RConn1
  Rigid Transform7/RConn1 -- Body/RConn1
